simulink model "Vienna_OCC"  (R2014b)
settings: Solver=ode45  StartTime=0.0  StopTime=0.2  FixedStep=1e-6  RelTol=1e-3
libraries: powerlib x29, powerlib_meascontrol x3, simulink x1
settings Model: Creator=rainman  LastModifiedBy=xh

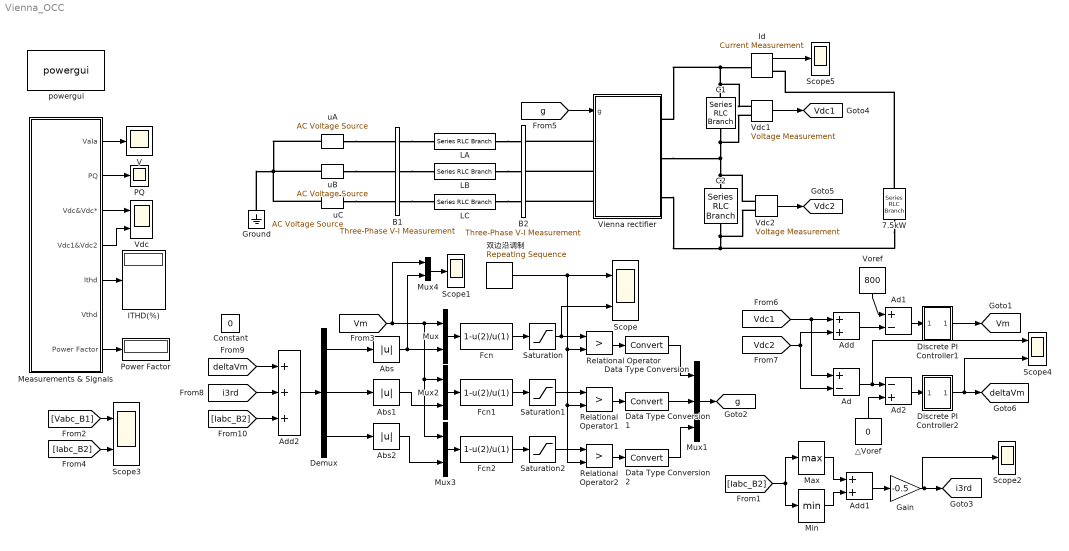
== system Vienna_OCC ==
  7.5kW : powerlib/Elements/Series RLC Branch  LConnTagsString=__new0  RConnTagsString=__new0  BranchType=R  Resistance=85.33  Inductance=1e-3  SetiL0=off  InitialCurrent=0  Capacitance=1e-6  Setx0=off  InitialVoltage=0  Measurements=None
  Abs : Abs
  Abs1 : Abs
  Abs2 : Abs
  Ad : Sum  Inputs=+-
  Ad1 : Sum  Inputs=+-
  Ad2 : Sum  Inputs=-+
  Add : Sum
  Add1 : Sum
  Add2 : Sum  Inputs=+++
  B1 : powerlib/Measurements/Three-Phase V-I Measurement  VoltageMeasurement=phase-to-ground  SetLabelV=on  LabelV=Vabc_B1  Vpu=off  VpuLL=off  CurrentMeasurement=no  SetLabelI=off  LabelI=Iabc_B1  Ipu=off  Pbase=100e6  Vbase=500e3  OutputType=Complex  PhasorSimulation=off  PSBequivalent=0
  B2 : powerlib/Measurements/Three-Phase V-I Measurement  VoltageMeasurement=no  SetLabelV=off  LabelV=Vabc_B1  Vpu=off  VpuLL=off  CurrentMeasurement=yes  SetLabelI=on  LabelI=Iabc_B2  Ipu=off  Pbase=100e6  Vbase=500e3  OutputType=Complex  PhasorSimulation=off  PSBequivalent=0
  C1 : powerlib/Elements/Series RLC Branch  LConnTagsString=__new0  RConnTagsString=__new0  BranchType=C  Resistance=1  Inductance=1e-3  SetiL0=off  InitialCurrent=0  Capacitance=850e-06  Setx0=off  InitialVoltage=0  Measurements=None
  C2 : powerlib/Elements/Series RLC Branch  LConnTagsString=__new0  RConnTagsString=__new0  BranchType=C  Resistance=1  Inductance=1e-3  SetiL0=off  InitialCurrent=0  Capacitance=850e-06  Setx0=off  InitialVoltage=0  Measurements=None
  Constant : Constant  Value=0
  Data Type Conversion : DataTypeConversion
  Data Type Conversion1 : DataTypeConversion
  Data Type Conversion2 : DataTypeConversion
  Demux : Demux  Outputs=3
  Discrete PI Controller1 : Subsystem  DialogController=POWERSYS.PowerSysDialog  mask(Discrete PI Controller){Kp=0.1, Ki=20, Par_Limits=[400 0], Init=0, Ts=1e-6}
      mask prompts: Kp "Proportional gain (Kp):"; Ki "Integral gain (Ki):"; Par_Limits "Output limits: [ Upper   Lower ]"; Init "Output initial value:"; Ts "Sample time:"
      mask help: This block implements a discrete PI controller.
      mask init:
      | UpperLimit=Par_Limits(1);
      | LowerLimit=Par_Limits(2);
      | power_initmask();
      mask Display: disp('PI');
  Discrete PI Controller2 : Subsystem  DialogController=POWERSYS.PowerSysDialog  mask(Discrete PI Controller){Kp=1, Ki=20, Par_Limits=[400 -400], Init=0, Ts=1e-6}
      mask prompts: Kp "Proportional gain (Kp):"; Ki "Integral gain (Ki):"; Par_Limits "Output limits: [ Upper   Lower ]"; Init "Output initial value:"; Ts "Sample time:"
      mask help: This block implements a discrete PI controller.
      mask init:
      | UpperLimit=Par_Limits(1);
      | LowerLimit=Par_Limits(2);
      | power_initmask();
      mask Display: disp('PI');
  Fcn : Fcn  Expr=1-u(2)/u(1)
  Fcn1 : Fcn  Expr=1-u(2)/u(1)
  Fcn2 : Fcn  Expr=1-u(2)/u(1)
  Gain : Gain  Gain=-0.5
  Ground : powerlib/Elements/Ground  LConnTagsString=a
  ITHD(%) : Display
      settings: Format=bank
  Id : powerlib/Measurements/Current Measurement  PhasorSimulation=off  OutputType=Complex  PSBequivalent=0
  LA : powerlib/Elements/Series RLC Branch  LConnTagsString=__new0  RConnTagsString=__new0  BranchType=RL  Resistance=0.1  Inductance=3e-3  SetiL0=off  InitialCurrent=0  Capacitance=1e-6  Setx0=off  InitialVoltage=0  Measurements=None
  LB : powerlib/Elements/Series RLC Branch  LConnTagsString=__new0  RConnTagsString=__new0  BranchType=RL  Resistance=0.1  Inductance=3e-3  SetiL0=off  InitialCurrent=0  Capacitance=1e-6  Setx0=off  InitialVoltage=0  Measurements=None
  LC : powerlib/Elements/Series RLC Branch  LConnTagsString=__new0  RConnTagsString=__new0  BranchType=RL  Resistance=0.1  Inductance=3e-3  SetiL0=off  InitialCurrent=0  Capacitance=1e-6  Setx0=off  InitialVoltage=0  Measurements=None
  Max : MinMax  Function=max
  Measurements & Signals : Subsystem
  Min : MinMax
  Mux{,2..4} (4 alike) : Mux  Inputs=2
  Mux1 : Mux  Inputs=3
  PQ : Scope
      settings: YMin=0  YMax=1000
  Power Factor : Display
  Relational Operator : RelationalOperator  Operator=>  OutDataTypeStr=boolean
  Relational Operator1 : RelationalOperator  Operator=>  OutDataTypeStr=boolean
  Relational Operator2 : RelationalOperator  Operator=>  OutDataTypeStr=boolean
  Saturation : Saturate  UpperLimit=1  LowerLimit=0
  Saturation1 : Saturate  UpperLimit=1  LowerLimit=0
  Saturation2 : Saturate  UpperLimit=1  LowerLimit=0
  Scope : Scope  NumInputPorts=2
      settings: YMin=0~0  YMax=1~1  SaveName=ScopeData14
  Scope1 : Scope
      settings: YMin=-50  YMax=400  SaveName=ScopeData3
  Scope2 : Scope
      settings: YMax=35  SaveName=ScopeData4
  Scope3 : Scope  NumInputPorts=2
      settings: YMin=0~0  YMax=1000~250  SaveName=ScopeData5
  Scope4 : Scope  NumInputPorts=2
      settings: YMin=-5000~-5  YMax=30000~5  SaveName=ScopeData6
  Scope5 : Scope
      settings: YMin=-5000  YMax=30000  SaveName=ScopeData7
  V : Scope
      settings: YMin=-400  YMax=400
  Vdc : Scope  NumInputPorts=2
      settings: YMin=0~0  YMax=1000~500  SaveName=ScopeData2
  Vdc1 : powerlib/Measurements/Voltage Measurement  PhasorSimulation=off  OutputType=Complex  PSBequivalent=0
  Vdc2 : powerlib/Measurements/Voltage Measurement  PhasorSimulation=off  OutputType=Complex  PSBequivalent=0
  Vienna rectifier : Subsystem
  Voref : Constant  Value=800
  powergui : powerlib/powergui  Priority=2  SimulationMode=Discrete  SolverType=Tustin  SampleTime=1e-06  frequency=60  SPID=off  DisableSnubberDevices=off  DisableRonSwitches=off  DisableVfSwitches=off  SwTol=0  DisplayEquations=off  Interpol=off  methode=off  Ts=0  frequencyindice=0  Pbase=100e6  ErrMax=1e-4  Iterations=50  UnitsV=kV  UnitsW=MW  FunctionMessages=off  echomessages=off  HookPort=off  EnableUseOfTLC=off  x0status=blocks  RestoreLinks=warning  ResistiveCurrentMeasurement=off  Frange=logspace(0,3,50)  Ylog=off  Xlog=off  ShowGrid=off  save=off  variable=ZData  structure=SinCos  ZoomFFT=off  StartTime=0.02  cycles=4  DisplayStyle=1  fundamental=50  FreqAxis=off  MaxFrequency=4000  frequencyindicesteady=1  RmsSteady=2  display=off
  uA : powerlib/Electrical Sources/AC Voltage Source  Amplitude=220*sqrt(2)  Phase=0  Frequency=50  SampleTime=0  Measurements=None
  uB : powerlib/Electrical Sources/AC Voltage Source  Amplitude=220*sqrt(2)  Phase=-120  Frequency=50  SampleTime=0  Measurements=None
  uC : powerlib/Electrical Sources/AC Voltage Source  Amplitude=220*sqrt(2)  Phase=120  Frequency=50  SampleTime=0  Measurements=None
  △Voref : Constant  Value=0
  双边沿调制 : simulink/Sources/Repeating Sequence  rep_seq_t="[0  0.000025 0.00005]"  rep_seq_y=[0 1 0]
  tag scope: Vdc1=global, Vdc2=global, Vm=global, deltaVm=global, g=global, i3rd=global
  wires:
  Vdc1/1 -> [Vdc1]
  Id/1 -> Scope5/1
  Vdc2/1 -> [Vdc2]
  [Iabc_B2] -> Max/1, Min/1
  [Vm] -> Mux4/1, Mux3/1, Mux2/1, Mux/1
  Abs/1 -> Mux4/2, Mux/2
  Mux/1 -> Fcn/1
  Abs1/1 -> Mux2/2
  Abs2/1 -> Mux3/2
  Mux2/1 -> Fcn1/1
  Mux3/1 -> Fcn2/1
  Measurements & Signals/5(Ithd) -> ITHD(%)/1
  Measurements & Signals/2(PQ) -> PQ/1
  Measurements & Signals/3(Vdc&Vdc*) -> Vdc/1
  Measurements & Signals/4(Vdc1&Vdc2) -> Vdc/2
  Relational Operator/1 -> Data Type Conversion/1
  双边沿调制/1 -> Relational Operator/2, Relational Operator1/2, Relational Operator2/2, Scope/1
  Relational Operator1/1 -> Data Type Conversion1/1
  Data Type Conversion1/1 -> Mux1/2
  Relational Operator2/1 -> Data Type Conversion2/1
  Data Type Conversion/1 -> Mux1/1
  Data Type Conversion2/1 -> Mux1/3
  Demux/1 -> Abs/1
  Demux/2 -> Abs1/1
  Demux/3 -> Abs2/1
  Mux4/1 -> Scope1/1
  [Vabc_B1] -> Scope3/1
  [Iabc_B2] -> Scope3/2
  Fcn/1 -> Saturation/1
  Saturation/1 -> Scope/2, Relational Operator/1
  Fcn1/1 -> Saturation1/1
  Saturation1/1 -> Relational Operator1/1
  Fcn2/1 -> Saturation2/1
  Saturation2/1 -> Relational Operator2/1
  Measurements & Signals/1(VaIa) -> V/1
  Mux1/1 -> [g]
  [g] -> Vienna rectifier/1(g)
  Discrete PI Controller1/1(Out) -> [Vm]
  [Vdc1] -> Add/1, Ad/1
  [Vdc2] -> Add/2, Ad/2
  Add/1 -> Ad1/2
  Ad1/1 -> Discrete PI Controller1/1(Error)
  Voref/1 -> Ad1/1
  Ad/1 -> Scope4/1, Ad2/1
  △Voref/1 -> Ad2/2
  Ad2/1 -> Discrete PI Controller2/1(Error)
  Max/1 -> Add1/1
  Min/1 -> Add1/2
  Add1/1 -> Gain/1
  Gain/1 -> Scope2/1, [i3rd]
  Add2/1 -> Demux/1
  [Iabc_B2] -> Add2/3
  Measurements & Signals/7(Power Factor) -> Power Factor/1
  [i3rd] -> Add2/2
  Discrete PI Controller2/1(Out) -> Scope4/2, [deltaVm]
  [deltaVm] -> Add2/1
  connections:
  C1/LConn1 -- Vienna rectifier/RConn1 -- Id/LConn1 -- Vdc1/LConn1
  C2/RConn1 -- Vdc2/LConn2 -- 7.5kW/RConn1 -- Vienna rectifier/RConn3
  C1/RConn1 -- Vdc1/LConn2 -- Vienna rectifier/RConn2 -- C2/LConn1 -- Vdc2/LConn1
  Vienna rectifier/LConn1 -- B2/RConn1
  Vienna rectifier/LConn2 -- B2/RConn2
  Ground/LConn1 -- uC/LConn1 -- uB/LConn1 -- uA/LConn1
  B1/RConn3 -- LC/LConn1
  uA/RConn1 -- B1/LConn1
  LB/RConn1 -- B2/LConn2
  uB/RConn1 -- B1/LConn2
  uC/RConn1 -- B1/LConn3
  LA/RConn1 -- B2/LConn1
  LC/RConn1 -- B2/LConn3
  B1/RConn1 -- LA/LConn1
  Vienna rectifier/LConn3 -- B2/RConn3
  B1/RConn2 -- LB/LConn1
  7.5kW/LConn1 -- Id/RConn1

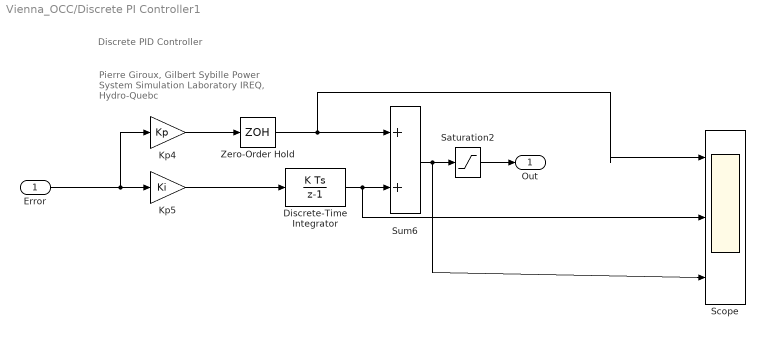
== system Vienna_OCC/Discrete PI Controller1 ==
  note: Discrete PID Controller
  note: Pierre Giroux, Gilbert Sybille
      | Power System Simulation Laboratory
      | IREQ, Hydro-Quebc
  Error : Inport  SampleTime=Ts
  Discrete-Time Integrator : DiscreteIntegrator  InitialCondition=Init  SampleTime=Ts  LimitOutput=on  UpperSaturationLimit=UpperLimit  LowerSaturationLimit=LowerLimit
  Kp4 : Gain  Gain=Kp  SampleTime=Ts  SaturateOnIntegerOverflow=on  OutDataTypeStr=Inherit: Same as input  ParamDataTypeStr=Inherit: Same as input
  Kp5 : Gain  Gain=Ki  SampleTime=Ts  SaturateOnIntegerOverflow=on  OutDataTypeStr=Inherit: Same as input  ParamDataTypeStr=Inherit: Same as input
  Saturation2 : Saturate  UpperLimit=UpperLimit  LowerLimit=LowerLimit  SampleTime=Ts
  Scope : Scope  NumInputPorts=3
      settings: YMin=-10~0~-10  YMax=20~20~30  SaveName=ScopeData17
  Sum6 : Sum  SampleTime=Ts  SaturateOnIntegerOverflow=on  InputSameDT=on  OutDataTypeStr=Inherit: Same as first input
  Zero-Order Hold : ZeroOrderHold  SampleTime=Ts
  Out : Outport  SampleTime=Ts  InitialOutput=0
  wires:
  Zero-Order Hold/1 -> Scope/1, Sum6/1
  Saturation2/1 -> Out/1
  Discrete-Time Integrator/1 -> Scope/2, Sum6/2
  Kp4/1 -> Zero-Order Hold/1
  Kp5/1 -> Discrete-Time Integrator/1
  Sum6/1 -> Scope/3, Saturation2/1
  Error/1 -> Kp5/1, Kp4/1

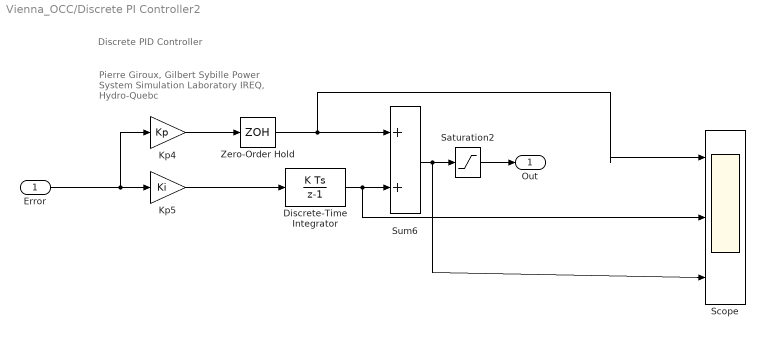
== system Vienna_OCC/Discrete PI Controller2 ==
  note: Pierre Giroux, Gilbert Sybille
      | Power System Simulation Laboratory
      | IREQ, Hydro-Quebc
  note: Discrete PID Controller
  Error : Inport  SampleTime=Ts
  Discrete-Time Integrator : DiscreteIntegrator  InitialCondition=Init  SampleTime=Ts  LimitOutput=on  UpperSaturationLimit=UpperLimit  LowerSaturationLimit=LowerLimit
  Kp4 : Gain  Gain=Kp  SampleTime=Ts  SaturateOnIntegerOverflow=on  OutDataTypeStr=Inherit: Same as input  ParamDataTypeStr=Inherit: Same as input
  Kp5 : Gain  Gain=Ki  SampleTime=Ts  SaturateOnIntegerOverflow=on  OutDataTypeStr=Inherit: Same as input  ParamDataTypeStr=Inherit: Same as input
  Saturation2 : Saturate  UpperLimit=UpperLimit  LowerLimit=LowerLimit  SampleTime=Ts
  Scope : Scope  NumInputPorts=3
      settings: YMin=-10~0~-10  YMax=20~20~30  SaveName=ScopeData17
  Sum6 : Sum  SampleTime=Ts  SaturateOnIntegerOverflow=on  InputSameDT=on  OutDataTypeStr=Inherit: Same as first input
  Zero-Order Hold : ZeroOrderHold  SampleTime=Ts
  Out : Outport  SampleTime=Ts  InitialOutput=0
  wires:
  Error/1 -> Kp4/1, Kp5/1
  Sum6/1 -> Saturation2/1, Scope/3
  Kp5/1 -> Discrete-Time Integrator/1
  Kp4/1 -> Zero-Order Hold/1
  Discrete-Time Integrator/1 -> Sum6/2, Scope/2
  Saturation2/1 -> Out/1
  Zero-Order Hold/1 -> Sum6/1, Scope/1

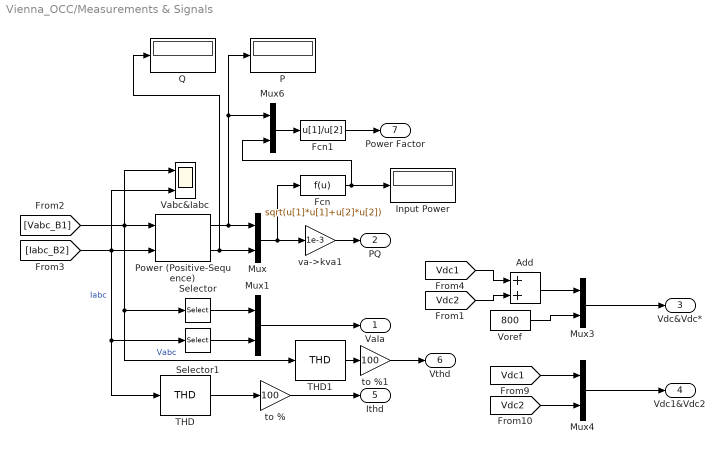
== system Vienna_OCC/Measurements & Signals ==
  Add : Sum
  Fcn : Fcn  Expr=sqrt(u[1]*u[1]+u[2]*u[2])
  Fcn1 : Fcn  Expr=u[1]/u[2]
  Input Power : Display
      settings: Format=bank
  Mux{,1,3..4,6} (5 alike) : Mux  Inputs=2
  P : Display
      settings: Format=bank
  Power (Positive-Sequence) : powerlib_meascontrol/Measurements/Power (Positive-Sequence)  Freq=50  Vinit=[280 0]  Iinit=[10 0]  Ts=1e-6
  Q : Display
      settings: Format=bank
  Selector : Selector  InputPortWidth=3
  Selector1 : Selector  InputPortWidth=3
  THD : powerlib_meascontrol/Measurements/THD  Freq=50  Ts=1e-6
  THD1 : powerlib_meascontrol/Measurements/THD  Freq=50  Ts=1e-6
  Vabc&Iabc : Scope  NumInputPorts=2
      settings: YMin=-5~-5  YMax=5~5  SaveName=ScopeData31
  Voref : Constant  Value=800
  to % : Gain  Gain=100
  to %1 : Gain  Gain=100
  va->kva1 : Gain  Gain=1e-3
  VaIa : Outport
  PQ : Outport  Port=2
  Vdc&Vdc* : Outport  Port=3
  Vdc1&Vdc2 : Outport  Port=4
  Ithd : Outport  Port=5
  Vthd : Outport  Port=6
  Power Factor : Outport  Port=7
  wires:
  [Vabc_B1] -> THD1/1, Selector/1, Vabc&Iabc/1, Power (Positive-Sequence)/1  "Vabc"
  [Iabc_B2] -> Vabc&Iabc/2, THD/1, Selector1/1, Power (Positive-Sequence)/2  "Iabc"
  Power (Positive-Sequence)/1 -> P/1, Mux6/1, Mux/1
  Power (Positive-Sequence)/2 -> Mux/2, Q/1
  Mux/1 -> Fcn/1, va->kva1/1
  va->kva1/1 -> PQ/1
  Mux1/1 -> VaIa/1
  Voref/1 -> Mux3/2
  Selector1/1 -> Mux1/2
  Selector/1 -> Mux1/1
  THD/1 -> to %/1
  to %/1 -> Ithd/1
  Fcn/1 -> Mux6/2, Input Power/1
  [Vdc1] -> Mux4/1
  [Vdc2] -> Mux4/2
  Mux3/1 -> Vdc&Vdc*/1
  Mux4/1 -> Vdc1&Vdc2/1
  Fcn1/1 -> Power Factor/1
  Mux6/1 -> Fcn1/1
  THD1/1 -> to %1/1
  to %1/1 -> Vthd/1
  [Vdc1] -> Add/1
  [Vdc2] -> Add/2
  Add/1 -> Mux3/1

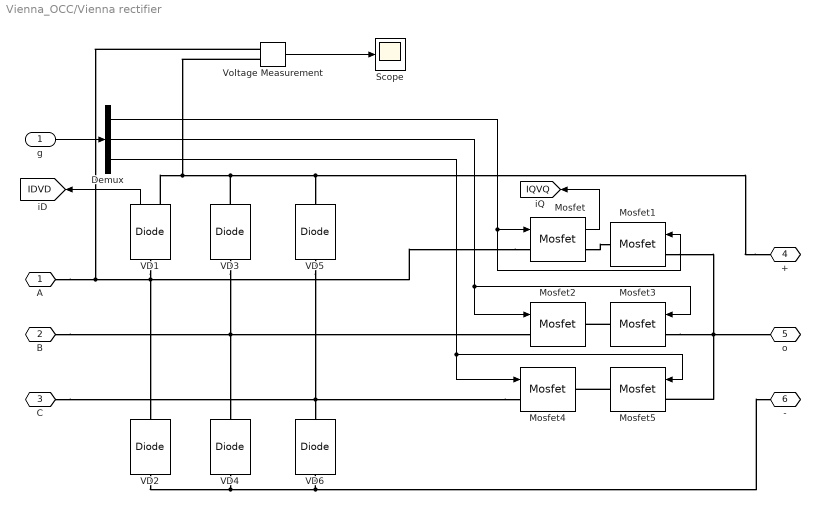
== system Vienna_OCC/Vienna rectifier ==
  g : Inport
  Demux : Demux  Outputs=3
  Mosfet : powerlib/Power Electronics/Mosfet  Ron=0.1  Lon=0  Rd=0.01  Vfd=0  IC=0  Rs=1e5  Cs=inf  Measurements=on
  Mosfet{1..5} (5 alike) : powerlib/Power Electronics/Mosfet  Ron=0.1  Lon=0  Rd=0.01  Vfd=0  IC=0  Rs=1e5  Cs=inf  Measurements=off
  Scope : Scope
      settings: SaveName=ScopeData18
  VD1 : powerlib/Power Electronics/Diode  Ron=0.001  Lon=0  Vf=0.8  IC=0  UseSnubber=off  Rs=500  Cs=250e-9  Measurements=on
  VD{2..6} (5 alike) : powerlib/Power Electronics/Diode  Ron=0.001  Lon=0  Vf=0.8  IC=0  UseSnubber=off  Rs=500  Cs=250e-9  Measurements=off
  Voltage Measurement : powerlib/Measurements/Voltage Measurement  PhasorSimulation=off  OutputType=Complex  PSBequivalent=0
  A : PMIOPort  Port=1  Side=Left
  B : PMIOPort  Port=2  Side=Left
  C : PMIOPort  Port=3  Side=Left
  + : PMIOPort  Port=4  Side=Right
  o : PMIOPort  Port=5  Side=Right
  - : PMIOPort  Port=6  Side=Right
  tag scope: IDVD=global, IQVQ=global
  wires:
  g/1 -> Demux/1
  Demux/1 -> Mosfet1/1, Mosfet/1
  Demux/2 -> Mosfet3/1, Mosfet2/1
  Demux/3 -> Mosfet5/1, Mosfet4/1
  VD1/1 -> [IDVD]
  Mosfet/1 -> [IQVQ]
  Voltage Measurement/1 -> Scope/1
  connections:
  Mosfet4/LConn1 -- VD6/RConn1 -- VD5/LConn1 -- C/RConn1
  VD3/LConn1 -- VD4/RConn1 -- B/RConn1 -- Mosfet2/LConn1
  Mosfet/LConn1 -- Voltage Measurement/LConn1 -- A/RConn1 -- VD2/RConn1 -- VD1/LConn1
  +/RConn1 -- VD5/RConn1 -- Voltage Measurement/LConn2 -- VD1/RConn1 -- VD3/RConn1
  VD6/LConn1 -- -/RConn1 -- VD2/LConn1 -- VD4/LConn1
  Mosfet3/LConn1 -- Mosfet1/LConn1 -- Mosfet5/LConn1 -- o/RConn1
  Mosfet3/RConn1 -- Mosfet2/RConn1
  Mosfet5/RConn1 -- Mosfet4/RConn1
  Mosfet/RConn1 -- Mosfet1/RConn1
